simulink model "qpsk_const"  (R2018b)
settings: Solver=VariableStepAuto  StartTime=0.0  StopTime=10.0  RelTol=1e-3
libraries: commrandsrc3 x1
settings Model: Creator=DSP_27  LastModifiedBy=DSP_27

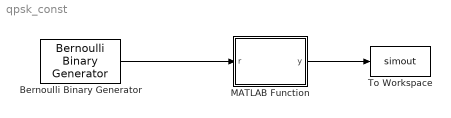
== system qpsk_const ==
  Bernoulli Binary Generator : commrandsrc3/Bernoulli Binary Generator  ProbabilityOfZero=0.5  SeedSource=Auto  Seed=0  SampleTime=1  SamplesPerFrame=10000  OutputDataType=double  SimulateUsing=Interpreted execution
  MATLAB Function : MATLAB Function  TreatAsAtomicUnit=on
  To Workspace : ToWorkspace  VariableName=simout  SaveFormat=Timeseries  SampleTime=-1
  wires:
  Bernoulli Binary Generator/1 -> MATLAB Function/1(r)
  MATLAB Function/1(y) -> To Workspace/1

== matlab function qpsk_const/MATLAB Function ==
  data: r input; y output
function y = fcn(r)
for i=1:2:N                     %converted to bpsk
    
        if((r(i)==0)&&(r(i+1)==0)) 
            r1(k) = 1+1j;
        
        elseif((r(i)==0)&&(r(i+1)==1))
            r1(k) = -1+1j;
        
        elseif((r(i)==1)&&(r(i+1)==0)) 
            r1(k) = -1-1j;
        
        elseif((r(i)==1)&&(r(i+1)==1)) 
            r1(k) = 1-1j;
           
        end
    k = k+1;

end
